simulink model "cpmphasetree"  (Simulink 6.0)
settings: Solver=ode3  SolverMode=SingleTasking  StartTime=0.0  StopTime=10.0  RelTol=1e-3
PreLoadFcn:
  | % Parameters are initialized in the Model Workspace
model workspace: external: M-Code (data not in the file)
undefined symbols (not defined in the file or in its folder): figposition, samplespersymbol, slcm
libraries: commsink2 x4, commdigbbndcpm2 x1, commutil2 x1, commrandsrc2 x1, dspsigops x1
CloseFcn:
  | clear cpmSigsOut
settings Model: Creator=mclune  LastModifiedBy=fwei  ProdHWDeviceType=Specified
settings DataIOCC: LimitDataPoints=off  SaveOutput=off  SaveTime=off  SignalLoggingName=cpmSigsOut
settings OptimizationCC: BlockReduction=off  BooleanDataType=off
settings DebuggingCC: CheckExecutionContextPreStartOutputMsg=on  CheckExecutionContextRuntimeOutputMsg=on  SolverPrmCheckMsg=none
settings HardwareCC: ProdHWDeviceType=Specified
settings ModelReferenceCC: UpdateModelReferenceTargets=IfOutOfDate
settings GRTTargetCC: LifeSpan=inf
settings SFSimCC: SFSimApplyToAllLibs=on  SFSimBuildMode=Incremental

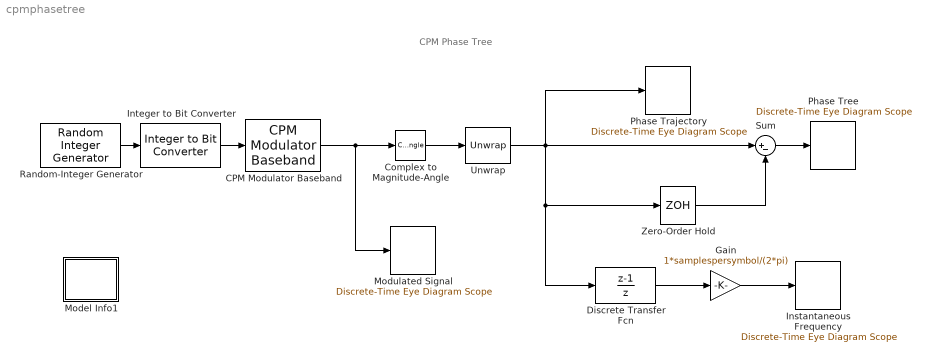
== system cpmphasetree ==
  note: CPM Phase Tree
  CPM Modulator Baseband : commdigbbndcpm2/CPM Modulator Baseband  Mnum=2  inputType=Bit  mappingType=Binary  modIdx=.5  pulseShape=Raised Cosine  BT=0.5  mainLobePulseLength=1  rollOff=0.2  pulseLength=1  preHistory=-1  phaseOffset=0  samplesPerSymbol=samplespersymbol
  Complex to Magnitude-Angle : ComplexToMagnitudeAngle  Output=Angle
  Discrete Transfer Fcn : DiscreteTransferFcn  Numerator=[1 -1]  Denominator=[1 0]  SampleTime=sampletime/samplespersymbol
  Gain : Gain  Gain=1*samplespersymbol/(2*pi)  SaturateOnIntegerOverflow=on
  Instantaneous Frequency : commsink2/Discrete-Time Eye Diagram Scope  Tag=EyeDiagram  sampPerSymb=samplespersymbol;  offsetEye=8  symbPerTrace=1  numTraces=48  numNewFrames=12  LineStyles=-  LineColors=b  dupPoints=on  fading=on  render=on  AxisGrid=on  yMin=-0.543093875812644  yMax=0.545562484339066  inphaseLabel=Instantaneous Frequency (MHz)  quadratureLabel=Quadrature Amplitude  openScopeAtSimStart=on  dispDiagram=In-phase Only  FrameNumber=off  FigPos=[576 445 403 350]  figTitle=Eye Diagram  block_type_=eye  numLinesMax=8
  Integer to Bit Converter : commutil2/Integer to Bit Converter  nbits=1
  Model Info1 : Subsystem  LoadFcn=slcm LoadBlock;  InitFcn=slcm('UpdateAllCMBlocksInThisModelInit')  EnableExecutionContextPropagation=on  mask(CMBlock){InitialSaveTempField=, InitialBlockCM=none, BlockCM=none, Frame=on, SaveTempField=, DisplayStringWithTags=Info, MaskDisplayString=Info, HorizontalTextAlignment=Center, LeftAlignmentValue=0.5, SourceBlockDiagram=cpmphasetree, TagMaxNumber=20, CMTag1=, CMTag2=, CMTag3=, CMTag4=, CMTag5=, CMTag6=, CMTag7=, CMTag8=, CMTag9=, CMTag10=, CMTag11=, CMTag12=, CMTag13=, CMTag14=, CMTag15=, CMTag16=, CMTag17=, CMTag18=, CMTag19=, CMTag20=}
      mask help: This block allows revision control information to be displayed within the model.
      settings: CopyFcn=slcm CopyBlock;  DeleteFcn=slcm Cancel;  PostSaveFcn=slcm('UpdateAllCMBlocksInThisModel')  NameChangeFcn=slcm Rename;  OpenFcn=commdemohelp;
      mask Display: text(str2num(LeftAlignmentValue), 0.5, MaskDisplayString, 'HorizontalAlignment', HorizontalTextAlignment)
  Modulated Signal : commsink2/Discrete-Time Eye Diagram Scope  Tag=EyeDiagram  sampPerSymb=samplespersymbol  offsetEye=8  symbPerTrace=2  numTraces=48  numNewFrames=12  LineStyles=-  LineColors=b  dupPoints=off  fading=on  render=on  AxisGrid=off  yMin=-1.1  yMax=1.105  inphaseLabel=In-phase Amplitude  quadratureLabel=Quadrature Amplitude  openScopeAtSimStart=off  dispDiagram=In-phase and Quadrature  FrameNumber=off  FigPos=figposition([5 60 30 30]);  figTitle=Eye Diagram  block_type_=eye  numLinesMax=8
  Phase Trajectory : commsink2/Discrete-Time Eye Diagram Scope  Tag=EyeDiagram  sampPerSymb=samplespersymbol  offsetEye=8  symbPerTrace=1  numTraces=48  numNewFrames=12  LineStyles=-  LineColors=r  dupPoints=off  fading=on  render=on  AxisGrid=on  yMin=-30  yMax=30  inphaseLabel=Phase Trajectory (rad.)  quadratureLabel=Quadrature Amplitude  openScopeAtSimStart=off  dispDiagram=In-phase Only  FrameNumber=off  FigPos=[58 52 288 250]  figTitle=Eye Diagram  block_type_=eye  numLinesMax=8
  Phase Tree : commsink2/Discrete-Time Eye Diagram Scope  Tag=EyeDiagram  sampPerSymb=samplespersymbol*3;  offsetEye=samplespersymbol*(3/2);  symbPerTrace=1  numTraces=16*3;  numNewFrames=samplespersymbol*(3/2);  LineMarkers=None  LineStyles=-  LineColors=m  dupPoints=off  fading=on  render=on  AxisGrid=on  yMin=-5.18091584979669  yMax=5.20446546729577  inphaseLabel=Phase Trajectory (rad.)  quadratureLabel=Quadrature Amplitude  openScopeAtSimStart=on  dispDiagram=In-phase Only  FrameNumber=off  FigPos=[576 45 346 301]  figTitle=Eye Diagram  block_type_=eye  numLinesMax=8
  Random-Integer Generator : commrandsrc2/Random Integer Generator  mul=2  seed=37  Ts=sampletime  frameBased=off  sampPerFrame=1  orient=off
  Sum : Sum  Inputs=|+-  SaturateOnIntegerOverflow=on  InputSameDT=on
  Unwrap : dspsigops/Unwrap  running=off  tol=pi
  Zero-Order Hold : ZeroOrderHold  SampleTime=1*sampletime*3
  wires:
  Complex to Magnitude-Angle/1 -> Unwrap/1
  Unwrap/1 -> Zero-Order Hold/1, Discrete Transfer Fcn/1, Sum/1, Phase Trajectory/1
  Zero-Order Hold/1 -> Sum/2
  Sum/1 -> Phase Tree/1
  Random-Integer Generator/1 -> Integer to Bit Converter/1
  Integer to Bit Converter/1 -> CPM Modulator Baseband/1
  CPM Modulator Baseband/1 -> Complex to Magnitude-Angle/1, Modulated Signal/1
  Discrete Transfer Fcn/1 -> Gain/1
  Gain/1 -> Instantaneous Frequency/1

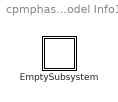
== system cpmphasetree/Model Info1 ==
  EmptySubsystem : Subsystem  EnableExecutionContextPropagation=on

== system cpmphasetree/Model Info1/EmptySubsystem ==
